simulink model "ltspidservo"  (Simulink 7.8)
settings: Solver=ode1  StartTime=0.0  StopTime=stoptime  FixedStep=(1/10000)  RelTol=1e-3
values from neighbouring files (symbols this model uses):
  Ap = A(1:4,1:4)    [GLTSsys.m]
  Ayaw = A(5:8,5:8)    [GLTSsys.m]
  Bp = B(1:4)'    [GLTSsys.m]
  Byaw = B(13:16)'    [GLTSsys.m]
  Cp = C(1:4)    [GLTSsys.m]
  Cyaw = [C(10) C(12) C(14) C(16)]    [GLTSsys.m]
  dt = 0.0001    [main.m]
  Gp = G(1:4,2)    [GLTSsys.m]
  Gyaw = G(5:8,6)    [GLTSsys.m]
  W = (1e-3)*eye(ny)    [KalmanEstimator.m]    (also in main.m = (1e-4)*eye(ny))
libraries: simulink x2
settings Model: Creator=Firdous  LastModifiedBy=Firdous
settings DataIOCC: LimitDataPoints=off

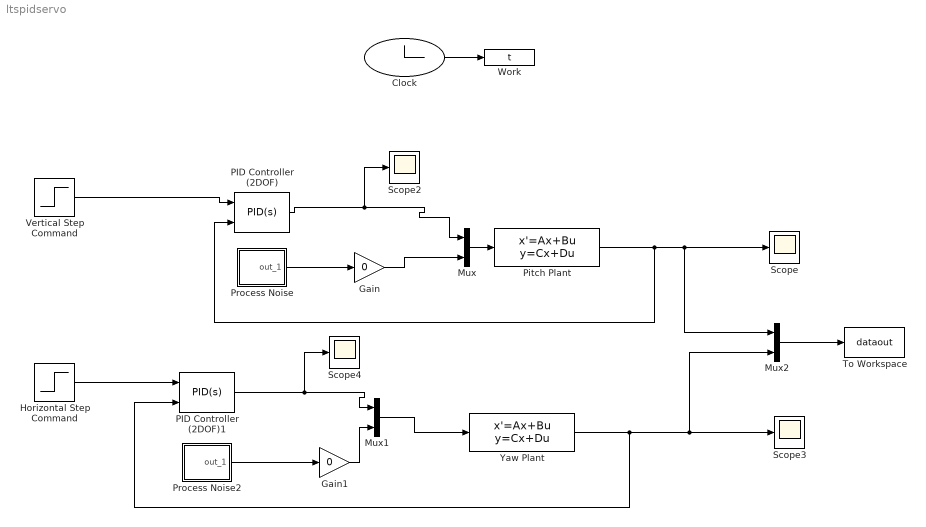
== system ltspidservo ==
  Clock : Clock
  Gain : Gain  Gain=0
  Gain1 : Gain  Gain=0
  Horizontal Step Command : Step  Time=0  After=15.15  SampleTime=0
  Mux : Mux  Inputs=2
  Mux1 : Mux  Inputs=2
  Mux2 : Mux  Inputs=2
  PID Controller (2DOF) : simulink/Continuous/PID Controller (2DOF)  Controller=PID  TimeDomain=Continuous-time  SampleTime=1  IntegratorMethod=Forward Euler  FilterMethod=Forward Euler  Form=Parallel  P=0.0058  I=7.009  D=0.0422  N=3.2773  b=1  c=1  InitialConditionSource=internal  InitialConditionForIntegrator=0  InitialConditionForFilter=0  ExternalReset=none  LimitOutput=on  UpperSaturationLimit=0.5  LowerSaturationLimit=-0.5  LinearizeAsGain=off  AntiWindupMode=none  Kb=1  TrackingMode=off  Kt=1  PParamMin=[]  PParamMax=[]  IParamMin=[]  IParamMax=[]  DParamMin=[]  DParamMax=[]  NParamMin=[]  NParamMax=[]  bParamMin=[]  bParamMax=[]  cParamMin=[]  cParamMax=[]  KbParamMin=[]  KbParamMax=[]  KtParamMin=[]  KtParamMax=[]  POutMin=[]  POutMax=[]  IOutMin=[]  IOutMax=[]  DOutMin=[]  DOutMax=[]  NOutMin=[]  NOutMax=[]  bOutMin=[]  bOutMax=[]  cOutMin=[]  cOutMax=[]  KbOutMin=[]  KbOutMax=[]  KtOutMin=[]  KtOutMax=[]  IntegratorOutMin=[]  IntegratorOutMax=[]  FilterOutMin=[]  FilterOutMax=[]  SumOutMin=[]  SumOutMax=[]  Sum1OutMin=[]  Sum1OutMax=[]  Sum2OutMin=[]  Sum2OutMax=[]  Sum3OutMin=[]  Sum3OutMax=[]  SumI1OutMin=[]  SumI1OutMax=[]  SumI2OutMin=[]  SumI2OutMax=[]  SumI3OutMin=[]  SumI3OutMax=[]  SumDOutMin=[]  SumDOutMax=[]  SaturationOutMin=[]  SaturationOutMax=[]  IntegratorContinuousStateAttributes=''  IntegratorStateMustResolveToSignalObject=off  IntegratorRTWStateStorageClass=Auto  FilterContinuousStateAttributes=''  FilterStateMustResolveToSignalObject=off  FilterRTWStateStorageClass=Auto
  PID Controller (2DOF)1 : simulink/Continuous/PID Controller (2DOF)  Controller=PID  TimeDomain=Continuous-time  SampleTime=1  IntegratorMethod=Forward Euler  FilterMethod=Forward Euler  Form=Parallel  P=0.0065  I=0.00012  D=0.0357  N=4.8923  b=1  c=1  InitialConditionSource=internal  InitialConditionForIntegrator=0  InitialConditionForFilter=0  ExternalReset=none  LimitOutput=on  UpperSaturationLimit=0.5  LowerSaturationLimit=-0.5  LinearizeAsGain=off  AntiWindupMode=none  Kb=1  TrackingMode=off  Kt=1  PParamMin=[]  PParamMax=[]  IParamMin=[]  IParamMax=[]  DParamMin=[]  DParamMax=[]  NParamMin=[]  NParamMax=[]  bParamMin=[]  bParamMax=[]  cParamMin=[]  cParamMax=[]  KbParamMin=[]  KbParamMax=[]  KtParamMin=[]  KtParamMax=[]  POutMin=[]  POutMax=[]  IOutMin=[]  IOutMax=[]  DOutMin=[]  DOutMax=[]  NOutMin=[]  NOutMax=[]  bOutMin=[]  bOutMax=[]  cOutMin=[]  cOutMax=[]  KbOutMin=[]  KbOutMax=[]  KtOutMin=[]  KtOutMax=[]  IntegratorOutMin=[]  IntegratorOutMax=[]  FilterOutMin=[]  FilterOutMax=[]  SumOutMin=[]  SumOutMax=[]  Sum1OutMin=[]  Sum1OutMax=[]  Sum2OutMin=[]  Sum2OutMax=[]  Sum3OutMin=[]  Sum3OutMax=[]  SumI1OutMin=[]  SumI1OutMax=[]  SumI2OutMin=[]  SumI2OutMax=[]  SumI3OutMin=[]  SumI3OutMax=[]  SumDOutMin=[]  SumDOutMax=[]  SaturationOutMin=[]  SaturationOutMax=[]  IntegratorContinuousStateAttributes=''  IntegratorStateMustResolveToSignalObject=off  IntegratorRTWStateStorageClass=Auto  FilterContinuousStateAttributes=''  FilterStateMustResolveToSignalObject=off  FilterRTWStateStorageClass=Auto
  Pitch Plant : StateSpace  A=Ap  B=[Bp Gp]  C=Cp  D=zeros(1,2)  X0=[2 0 0 0]
  Process Noise : Subsystem  mask(Continuous White Noise.){Cov=W, Ts=dt, seed=[23341]}
      mask prompts: Cov "Noise Variance:"; Ts "Sample Time:"
      mask help:
      | White noise for continuous (s-domain) systems.
      | Band-limited using zero-order-hold.
      mask Help: Implemented using white noise into Zero Order Hold block. For faster simulation set sample time to highest value possible but in accordance with the fastest dynamics of system.
      mask Display: plot(1:20,rand(size(1:20)))
  Process Noise2 : Subsystem  mask(Continuous White Noise.){Cov=W, Ts=dt, seed=[23341]}
      mask prompts: Cov "Noise Variance:"; Ts "Sample Time:"
      mask help:
      | White noise for continuous (s-domain) systems.
      | Band-limited using zero-order-hold.
      mask Help: Implemented using white noise into Zero Order Hold block. For faster simulation set sample time to highest value possible but in accordance with the fastest dynamics of system.
      mask Display: plot(1:20,rand(size(1:20)))
  Scope{,2..4} (4 alike) : Scope
      Scope settings: YMin=-6500  YMax=2000
      Scope2 settings: YMin=17  YMax=31  SaveName=ScopeData2
      Scope3 settings: YMin=14.2  YMax=15.9  SaveName=ScopeData3
      Scope4 settings: YMin=17  YMax=31  SaveName=ScopeData4
  To Workspace : ToWorkspace  VariableName=dataout  SampleTime=-1  SaveFormat=Array
  Vertical Step Command : Step  Time=0  After=15.15  SampleTime=0
  Work : ToWorkspace  VariableName=t  SaveFormat=Array
  Yaw Plant : StateSpace  A=Ayaw  B=[Byaw Gyaw]  C=Cyaw  D=zeros(1,2)  X0=[2 0 0 0]
  wires:
  Clock/1 -> Work/1
  Pitch Plant/1 -> PID Controller (2DOF)/2, Scope/1, Mux2/1
  Vertical Step Command/1 -> PID Controller (2DOF)/1
  Mux/1 -> Pitch Plant/1
  PID Controller (2DOF)/1 -> Scope2/1, Mux/1
  Process Noise/1(out_1) -> Gain/1
  Gain/1 -> Mux/2
  Yaw Plant/1 -> PID Controller (2DOF)1/2, Scope3/1, Mux2/2
  Horizontal Step Command/1 -> PID Controller (2DOF)1/1
  Mux1/1 -> Yaw Plant/1
  PID Controller (2DOF)1/1 -> Scope4/1, Mux1/1
  Process Noise2/1(out_1) -> Gain1/1
  Gain1/1 -> Mux1/2
  Mux2/1 -> To Workspace/1

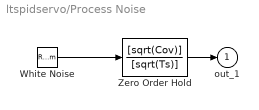
== system ltspidservo/Process Noise ==
  White Noise : RandomNumber  Seed=seed  SampleTime=dt
  Zero Order Hold : DiscreteTransferFcn  Numerator=[sqrt(Cov)]  Denominator=[sqrt(Ts)]  SampleTime=Ts
  out_1 : Outport
  wires:
  Zero Order Hold/1 -> out_1/1
  White Noise/1 -> Zero Order Hold/1

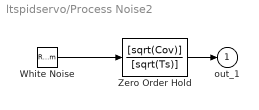
== system ltspidservo/Process Noise2 ==
  White Noise : RandomNumber  Seed=seed  SampleTime=dt
  Zero Order Hold : DiscreteTransferFcn  Numerator=[sqrt(Cov)]  Denominator=[sqrt(Ts)]  SampleTime=Ts
  out_1 : Outport
  wires:
  Zero Order Hold/1 -> out_1/1
  White Noise/1 -> Zero Order Hold/1
